simulink model "Traslacional"  (R2023b)
settings: Solver=VariableStepAuto  StartTime=0.0  StopTime=10.0  RelTol=1e-3
undefined symbols (not defined in the file): b1, k1, k2, m1, m2
settings Model: Creator=USER  LastModifiedBy=USER

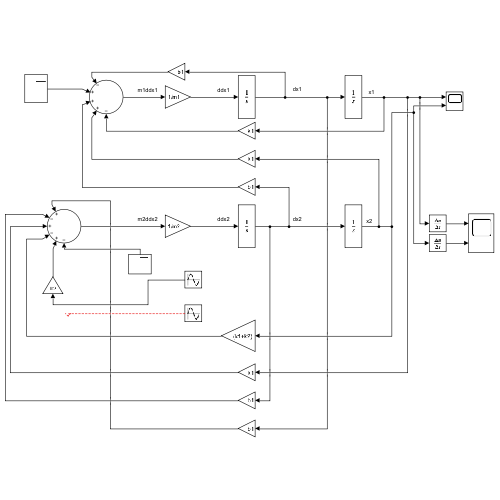
[thumbnail: Simulink's stored preview of the top-level diagram]
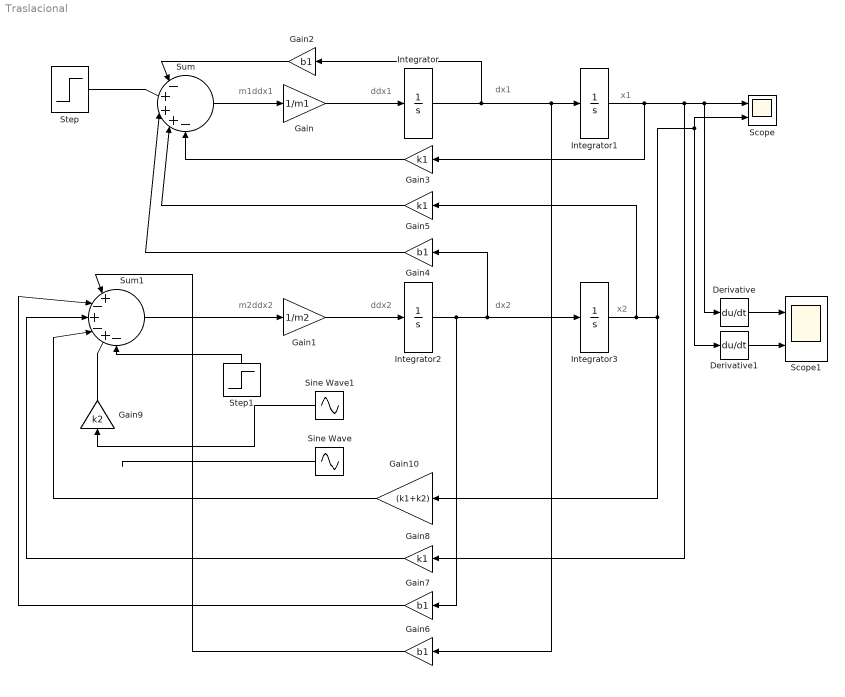
== system Traslacional ==
  note: x1
  note: dx1
  note: ddx1
  note: m1ddx1
  note: ddx2
  note: dx2
  note: x2
  note: m2ddx2
  Derivative : Derivative
  Derivative1 : Derivative
  Gain : Gain  Gain=1/m1
  Gain1 : Gain  Gain=1/m2
  Gain10 : Gain  Gain=(k1+k2)
  Gain{2,4,6..7} (4 alike) : Gain  Gain=b1
  Gain3 : Gain  Gain=k1
  Gain5 : Gain  Gain=k1
  Gain8 : Gain  Gain=k1
  Gain9 : Gain  Gain=k2
  Integrator{,1..3} (4 alike) : Integrator
  Scope : Scope  NumInputPorts=2
  Scope1 : Scope  NumInputPorts=2
  Sine Wave : Sin  Amplitude=0.05  Frequency=20*pi  SampleTime=0
  Sine Wave1 : Sin  Amplitude=0.05  Frequency=.5*pi  SampleTime=0
  Step : Step  Time=0  After=0  SampleTime=0
  Step1 : Step  Time=0  After=0  SampleTime=0
  Sum : Sum  Inputs=|-+++-
  Sum1 : Sum  Inputs=|+-+-+-
  wires:
  Gain/1 -> Integrator/1
  Sum/1 -> Gain/1
  Integrator/1 -> Gain6/1, Integrator1/1, Gain2/1
  Gain1/1 -> Integrator2/1
  Integrator2/1 -> Integrator3/1, Gain4/1, Gain7/1
  Integrator3/1 -> Scope/2, Derivative1/1, Gain10/1, Gain5/1
  Sum1/1 -> Gain1/1
  Step/1 -> Sum/2
  Gain2/1 -> Sum/1
  Gain3/1 -> Sum/5
  Gain4/1 -> Sum/3
  Gain5/1 -> Sum/4
  Gain6/1 -> Sum1/1
  Gain7/1 -> Sum1/2
  Gain8/1 -> Sum1/3
  Step1/1 -> Sum1/6
  Gain10/1 -> Sum1/4
  Gain9/1 -> Sum1/5
  Derivative/1 -> Scope1/1
  Integrator1/1 -> Derivative/1, Scope/1, Gain8/1, Gain3/1
  Derivative1/1 -> Scope1/2
  Sine Wave/1 -> ?
  Sine Wave1/1 -> Gain9/1
